simulink model "car1st"  (R2021b)
settings: Solver=VariableStepAuto  StartTime=0.0  StopTime=30  RelTol=1e-3
settings Model: Creator=minna  LastModifiedBy=minna

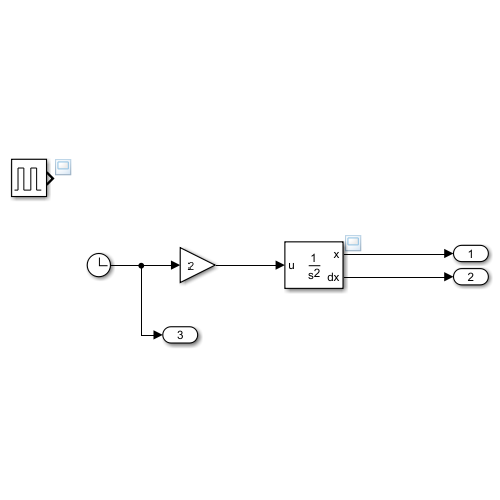
[thumbnail: Simulink's stored preview of the top-level diagram]
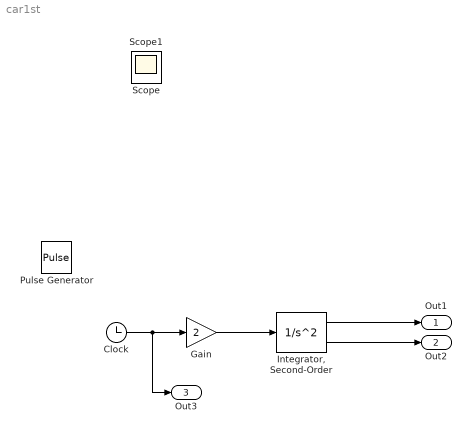
== system car1st ==
  Clock : Clock
  Gain : Gain  Gain=2
  "Integrator, Second-Order" : SecondOrderIntegrator
  Pulse Generator : DiscretePulseGenerator  PulseType=Time based  Period=10  PulseWidth=5
  Out1 : Outport
  Out2 : Outport  Port=2
  Out3 : Outport  Port=3
  Scope : Scope
  Scope1 : Scope
  wires:
  Gain/1 -> "Integrator, Second-Order"/1
  "Integrator, Second-Order"/1 -> Out1/1
  "Integrator, Second-Order"/2 -> Out2/1
  Clock/1 -> Out3/1, Gain/1
